simulink model "NPC_ANPC_Final_A"  (R2022b)
settings: Solver=ode4  StartTime=0.0  StopTime=1  FixedStep=1e-6  MaxStep=1e-4  RelTol=1e-3
InitFcn:
  | v=3000
  | r=0.000001
  | c=1000e-6
  | l=314
  | i=1000
  | r1=1000
  | t=1/3000
  | ma=2
  | f=2*pi*50
  | p1=(2*pi)/3
  | p2=-(2*pi)/3
libraries: spsIGBTDiodeLib x25, spsDiodeLib x19, simulink x12, spsSeriesRLCBranchLib x7, spsVoltageMeasurementLib x3, spsCurrentMeasurementLib x2, spsMeanLib x2, spspowerguiLib x2, spsPermanentMagnetSynchronousMachineLib x1, spsThreePhaseVIMeasurementLib x1, spsWindTurbineLib x1
settings Model: Creator=dell  LastModifiedBy=shubh
settings SolverCC: AlgebraicLoopSolver=TrustRegion
settings DataIOCC: ReturnWorkspaceOutputs=off
settings DebuggingCC: UnconnectedInputMsg=warning  UnconnectedOutputMsg=warning  UnconnectedLineMsg=warning  SFMachineParentedDataDiag=warning  ArithmeticOperatorsInVariantConditions=warning
settings ModelReferenceCC: EnableRefExpFcnMdlSchedulingChecks=on
settings SFSimCC: SimUseLocalCustomCode=off  CustomCodeUndefinedFunction=UseInterfaceOnly
settings RTWCC: RTWUseLocalCustomCode=off
settings CodeAppCC: StateflowObjectComments=on
settings SimscapeCC: SimscapeNormalizeSystem=off

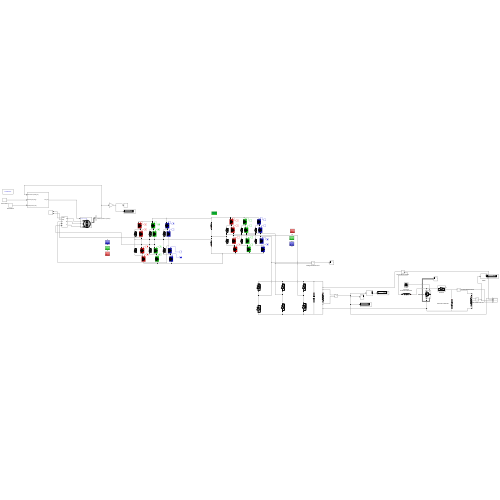
[thumbnail: Simulink's stored preview of the top-level diagram]
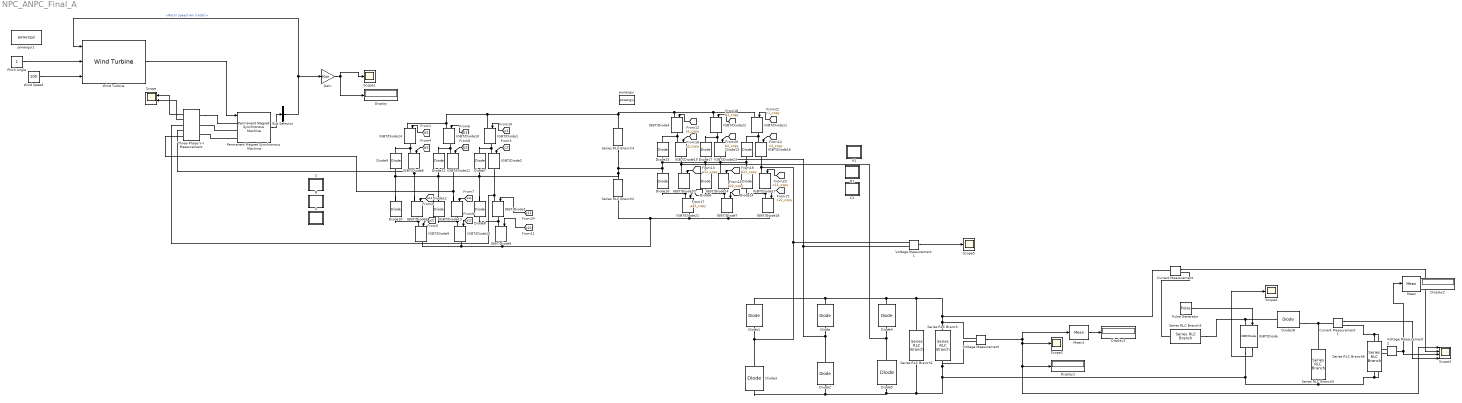
== system NPC_ANPC_Final_A ==
  A : Subsystem
  A1 : Subsystem
  B : Subsystem
  B1 : Subsystem
  Bus Selector : BusSelector  OutputSignals=Rotor speed wm (rad/s)
  C : Subsystem
  C1 : Subsystem
  Current Measurement : spsCurrentMeasurementLib/Current Measurement  PhasorSimulation=off  OutputType=Complex  PSBequivalent=0
  Current Measurement1 : spsCurrentMeasurementLib/Current Measurement  PhasorSimulation=off  OutputType=Complex  PSBequivalent=0
  Diode{,1..17} (18 alike) : spsDiodeLib/Diode  Ron=0.001  Lon=0  Vf=0.8  IC=0  UseSnubber=0  Rs=500  Cs=250e-9  Measurements=off
  Diode18 : spsDiodeLib/Diode  Ron=0.001  Lon=0  Vf=0.8  IC=0  UseSnubber=0  Rs=500  Cs=250e-9  Measurements=on
  Display{,1..3} (4 alike) : Display
  Gain : Gain  Gain=30/pi
  IGBT/Diode : spsIGBTDiodeLib/IGBT//Diode  Ron=1e-3  Rs=1e5  Cs=inf  Measurements=on
  IGBT/Diode{1..24} (24 alike) : spsIGBTDiodeLib/IGBT//Diode  Ron=1e-3  Rs=1e5  Cs=inf  Measurements=off
  Mean : spsMeanLib/Mean  Freq=60  Vinit=0  Ts=0
  Mean1 : spsMeanLib/Mean  Freq=60  Vinit=0  Ts=0
  Permanent Magnet Synchronous Machine : spsPermanentMagnetSynchronousMachineLib/Permanent Magnet Synchronous Machine  NbPhases=3  FluxDistribution=Sinusoidal  RotorType=Round  MechanicalLoad=Torque Tm  PresetModel=No  ShowDetailedParameters=on  MeasurementBus=off  Resistance=0.0485  Inductance=8.5e-3  dqInductances=[8.5e-3,8.5e-3]  La=0.000395  MachineConstant=Flux linkage established by magnets (V.s)  Flux=0.1194  VoltageCst=86.6271  TorqueCst=0.7164  Flat=120  Mechanical=[0.0027 0.0004924 4 0]  PolePairs=4  InitialConditions=[0,0, 0,0]  InitialConditions5ph=[0 0 0 0 0 0]  RefAngle=90 degrees behind phase A axis (modified Park)  IterativeDiscreteModel=Trapezoidal non iterative  TsBlock=-1  TsPowergui=0
  Pitch Angle : Constant
  Pulse Generator : DiscretePulseGenerator  PulseType=Time based  Amplitude=4  Period=1/5000  PulseWidth=60
  Scope : Scope  NumInputPorts=2
  Scope{1..2,4..5} (4 alike) : Scope
  Scope3 : Scope  NumInputPorts=4
  Series RLC Branch : spsSeriesRLCBranchLib/Series RLC Branch  LConnTagsString=__new0  RConnTagsString=__new0  BranchType=R  Resistance=10  Inductance=1e-3  SetiL0=off  InitialCurrent=0  Capacitance=1e-6  Setx0=off  InitialVoltage=0  Measurements=None
  Series RLC Branch1 : spsSeriesRLCBranchLib/Series RLC Branch  LConnTagsString=__new0  RConnTagsString=__new0  BranchType=C  Resistance=10  Inductance=10e-3  SetiL0=off  InitialCurrent=0  Capacitance=10e-3  Setx0=off  InitialVoltage=0  Measurements=None
  Series RLC Branch2 : spsSeriesRLCBranchLib/Series RLC Branch  LConnTagsString=__new0  RConnTagsString=__new0  BranchType=C  Resistance=1  Inductance=1e-3  SetiL0=off  InitialCurrent=0  Capacitance=5000e-6  Setx0=off  InitialVoltage=i  Measurements=None
  Series RLC Branch3 : spsSeriesRLCBranchLib/Series RLC Branch  LConnTagsString=__new0  RConnTagsString=__new0  BranchType=L  Resistance=1  Inductance=6e-3  SetiL0=off  InitialCurrent=0  Capacitance=1e-6  Setx0=off  InitialVoltage=0  Measurements=None
  Series RLC Branch4 : spsSeriesRLCBranchLib/Series RLC Branch  LConnTagsString=__new0  RConnTagsString=__new0  BranchType=C  Resistance=1  Inductance=1e-3  SetiL0=off  InitialCurrent=0  Capacitance=5000e-6  Setx0=off  InitialVoltage=i  Measurements=None
  Series RLC Branch5 : spsSeriesRLCBranchLib/Series RLC Branch  LConnTagsString=__new0  RConnTagsString=__new0  BranchType=C  Resistance=1  Inductance=6e-3  SetiL0=off  InitialCurrent=0  Capacitance=5000e-6  Setx0=off  InitialVoltage=0  Measurements=None
  Series RLC Branch6 : spsSeriesRLCBranchLib/Series RLC Branch  LConnTagsString=__new0  RConnTagsString=__new0  BranchType=R  Resistance=12.5  Inductance=6e-3  SetiL0=off  InitialCurrent=0  Capacitance=1e-6  Setx0=off  InitialVoltage=0  Measurements=None
  Three-Phase V-I Measurement : spsThreePhaseVIMeasurementLib/Three-Phase V-I Measurement  VoltageMeasurement=phase-to-phase  SetLabelV=off  LabelV=Vabc  Vpu=off  VpuLL=off  CurrentMeasurement=yes  SetLabelI=off  LabelI=Iabc  Ipu=off  Pbase=100e6  Vbase=500e3  OutputType=Complex  PhasorSimulation=off  PSBequivalent=0
  Voltage Measurement : spsVoltageMeasurementLib/Voltage Measurement  PhasorSimulation=off  OutputType=Complex  PSBequivalent=0
  Voltage Measurement1 : spsVoltageMeasurementLib/Voltage Measurement  PhasorSimulation=off  OutputType=Complex  PSBequivalent=0
  Voltage Measurement2 : spsVoltageMeasurementLib/Voltage Measurement  PhasorSimulation=off  OutputType=Complex  PSBequivalent=0
  Wind Speed : Constant  Value=100
  Wind Turbine : spsWindTurbineLib/Wind Turbine  Pnom=1.5e6  Pelec_base=1.5e6/0.9  wind_base=12  P_wind_base=0.73  speed_nom=1.2  pitch_angle=0  c1_c6="[0.51763          116          0.4            5           21     0.006795]"  cp_nom=0.48  lambda_nom=8.1
  powergui : spspowerguiLib/powergui  Priority=1  SimulationMode=Discrete  SampleTime=1e-6  frequency=60  Iterations=50  frequencyindice=0  Pbase=100e6  ErrMax=1e-4  UnitsV=kV  UnitsW=MW  buscounter=0  FunctionMessages=off  echomessages=off  EnableUseOfTLC=off  CurrentSourceSwitches=off  DisableSnubberDevices=off  DisableRonSwitches=off  DisableVfSwitches=off  DisplayEquations=off  AutomaticDiscreteSolvers=off  SolverType=Tustin/Backward Euler (TBE)  Interpol=off  ExternalGateDelay=off  methode=off  Ts=100  x0status=blocks  SPID=on  SwTol=0  HookPort=off  NonlinearTolerance=1e-4  nMaxIteration=100  ContinueOnMaxIteration=off  RestoreLinks=warning  ResistiveCurrentMeasurement=off  Frange=[0:2:500]  Ylog=off  Xlog=on  ShowGrid=off  save=off  variable=ZData  structure=d  ZoomFFT=off  StartTime=0.2  cycles=2  DisplayStyle=1  fundamental=50  FreqAxis=on  MaxFrequency=40000  frequencyindicesteady=1  RmsSteady=1  display=off
  powergui1 : spspowerguiLib/powergui  Priority=1  SimulationMode=Continuous  SampleTime=50e-6  frequency=60  Iterations=50  frequencyindice=0  Pbase=100e6  ErrMax=1e-4  UnitsV=kV  UnitsW=MW  buscounter=0  FunctionMessages=off  echomessages=off  EnableUseOfTLC=off  CurrentSourceSwitches=off  DisableSnubberDevices=off  DisableRonSwitches=off  DisableVfSwitches=off  DisplayEquations=off  AutomaticDiscreteSolvers=off  SolverType=Tustin/Backward Euler (TBE)  Interpol=off  ExternalGateDelay=off  methode=off  Ts=100  x0status=blocks  SPID=on  SwTol=0  HookPort=off  NonlinearTolerance=1e-4  nMaxIteration=100  ContinueOnMaxIteration=off  RestoreLinks=warning  ResistiveCurrentMeasurement=off  Frange=[0:2:500]  Ylog=off  Xlog=on  ShowGrid=off  save=off  variable=ZData  structure=0  ZoomFFT=off  StartTime=0.0  cycles=1  DisplayStyle=1  fundamental=60  FreqAxis=off  MaxFrequency=1000  frequencyindicesteady=1  RmsSteady=1  display=off
  wires:
  Gain/1 -> Display/1, Scope1/1
  Pitch Angle/1 -> Wind Turbine/2
  Bus Selector/1 -> Gain/1, Wind Turbine/1  "<Rotor speed wm (rad/s)>"
  Three-Phase V-I Measurement/1 -> Scope/1
  Wind Turbine/1 -> Permanent Magnet Synchronous Machine/1
  Permanent Magnet Synchronous Machine/1 -> Bus Selector/1
  Wind Speed/1 -> Wind Turbine/3
  Three-Phase V-I Measurement/2 -> Scope/2
  [c22_copy] -> IGBT/Diode18/1
  [c2_copy] -> IGBT/Diode16/1
  [c1_copy] -> IGBT/Diode11/1
  [c11_copy] -> IGBT/Diode17/1
  [b22_copy] -> IGBT/Diode7/1
  [b11_copy] -> IGBT/Diode24/1
  [b2_copy] -> IGBT/Diode23/1
  [b1_copy] -> IGBT/Diode22/1
  [a22_copy] -> IGBT/Diode21/1
  [a11_copy] -> IGBT/Diode20/1
  [a2_copy] -> IGBT/Diode19/1
  [a1_copy] -> IGBT/Diode4/1
  [c1] -> IGBT/Diode1/1
  [c2] -> IGBT/Diode2/1
  [c22] -> IGBT/Diode5/1
  [a22] -> IGBT/Diode9/1
  [a2] -> IGBT/Diode6/1
  [a11] -> IGBT/Diode8/1
  [b2] -> IGBT/Diode12/1
  [b1] -> IGBT/Diode10/1
  [b11] -> IGBT/Diode13/1
  [b22] -> IGBT/Diode15/1
  [c11] -> IGBT/Diode3/1
  [a1] -> IGBT/Diode14/1
  Voltage Measurement1/1 -> Scope5/1
  Mean/1 -> Display2/1
  IGBT/Diode/1 -> Scope4/1
  Pulse Generator/1 -> IGBT/Diode/1
  Voltage Measurement2/1 -> Mean/1, Scope3/3
  Mean1/1 -> Display3/1
  Current Measurement1/1 -> Scope3/4
  Current Measurement/1 -> Scope3/2
  Voltage Measurement/1 -> Scope3/1, Display1/1, Scope2/1, Mean1/1
  connections:
  Permanent Magnet Synchronous Machine/LConn2 -- Three-Phase V-I Measurement/LConn2
  Three-Phase V-I Measurement/LConn1 -- Permanent Magnet Synchronous Machine/LConn1
  Permanent Magnet Synchronous Machine/LConn3 -- Three-Phase V-I Measurement/LConn3
  IGBT/Diode19/LConn1 -- Diode15/RConn1 -- IGBT/Diode4/RConn1
  IGBT/Diode21/LConn1 -- Diode16/LConn1 -- IGBT/Diode20/RConn1
  IGBT/Diode23/LConn1 -- Diode17/RConn1 -- IGBT/Diode22/RConn1
  IGBT/Diode7/LConn1 -- Diode6/LConn1 -- IGBT/Diode24/RConn1
  IGBT/Diode16/LConn1 -- Diode13/RConn1 -- IGBT/Diode11/RConn1
  IGBT/Diode18/LConn1 -- Diode14/LConn1 -- IGBT/Diode17/RConn1
  Diode12/RConn1 -- Diode11/LConn1 -- Diode10/RConn1 -- Diode9/LConn1 -- Diode7/LConn1 -- Series RLC Branch4/LConn1 -- Diode16/RConn1 -- Diode15/LConn1 -- Diode6/RConn1 -- Diode17/LConn1 -- Diode14/RConn1 -- Diode13/LConn1 -- Series RLC Branch2/RConn1 -- Diode8/RConn1
  IGBT/Diode24/LConn1 -- IGBT/Diode23/RConn1 -- Voltage Measurement1/LConn2 -- Diode/LConn1 -- Diode2/RConn1
  IGBT/Diode15/RConn1 -- IGBT/Diode9/RConn1 -- IGBT/Diode5/RConn1 -- Series RLC Branch2/LConn1 -- IGBT/Diode21/RConn1 -- IGBT/Diode7/RConn1 -- IGBT/Diode18/RConn1
  IGBT/Diode10/LConn1 -- IGBT/Diode14/LConn1 -- IGBT/Diode1/LConn1 -- Series RLC Branch4/RConn1 -- IGBT/Diode4/LConn1 -- IGBT/Diode22/LConn1 -- IGBT/Diode11/LConn1
  Diode4/LConn1 -- IGBT/Diode20/LConn1 -- IGBT/Diode19/RConn1 -- Diode5/RConn1
  Diode8/LConn1 -- IGBT/Diode5/LConn1 -- IGBT/Diode3/RConn1
  Diode10/LConn1 -- IGBT/Diode9/LConn1 -- IGBT/Diode8/RConn1
  Diode12/LConn1 -- IGBT/Diode15/LConn1 -- IGBT/Diode13/RConn1
  IGBT/Diode14/RConn1 -- IGBT/Diode6/LConn1 -- Diode9/RConn1
  Diode11/RConn1 -- IGBT/Diode12/LConn1 -- IGBT/Diode10/RConn1
  Diode7/RConn1 -- IGBT/Diode2/LConn1 -- IGBT/Diode1/RConn1
  Three-Phase V-I Measurement/RConn1 -- IGBT/Diode3/LConn1 -- IGBT/Diode2/RConn1
  Series RLC Branch1/RConn1 -- Voltage Measurement/LConn2 -- Series RLC Branch/RConn1 -- Voltage Measurement2/LConn2 -- Series RLC Branch6/RConn1 -- Series RLC Branch5/RConn1 -- IGBT/Diode/RConn1 -- Diode5/LConn1 -- Diode3/LConn1 -- Diode2/LConn1
  Diode18/LConn1 -- Series RLC Branch3/LConn1 -- IGBT/Diode/LConn1
  Diode4/RConn1 -- Voltage Measurement/LConn1 -- Series RLC Branch/LConn1 -- Current Measurement/LConn1 -- Series RLC Branch1/LConn1 -- Diode1/RConn1 -- Diode/RConn1
  Series RLC Branch6/LConn1 -- Voltage Measurement2/LConn1 -- Current Measurement1/RConn1
  Current Measurement1/LConn1 -- Diode18/RConn1 -- Series RLC Branch5/LConn1
  Series RLC Branch3/RConn1 -- Current Measurement/RConn1
  IGBT/Diode13/LConn1 -- IGBT/Diode12/RConn1 -- Three-Phase V-I Measurement/RConn3
  IGBT/Diode8/LConn1 -- Three-Phase V-I Measurement/RConn2 -- IGBT/Diode6/RConn1
  Voltage Measurement1/LConn1 -- Diode1/LConn1 -- Diode3/RConn1 -- IGBT/Diode17/LConn1 -- IGBT/Diode16/RConn1

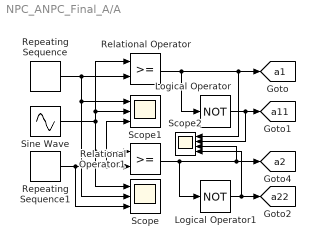
== system NPC_ANPC_Final_A/A ==
  Logical Operator : Logic  Operator=NOT  AllPortsSameDT=off  OutDataTypeStr=boolean
  Logical Operator1 : Logic  Operator=NOT  AllPortsSameDT=off  OutDataTypeStr=boolean
  Relational Operator : RelationalOperator  OutDataTypeStr=boolean  RndMeth=Simplest  InputSameDT=off
  Relational Operator1 : RelationalOperator  OutDataTypeStr=boolean  RndMeth=Simplest  InputSameDT=off
  Repeating Sequence : simulink/Sources/Repeating Sequence  rep_seq_t=[0 t/2 t]  rep_seq_y=[0 2 0]
  Repeating Sequence1 : simulink/Sources/Repeating Sequence  rep_seq_t=[0 t/2 t]  rep_seq_y=[-2 0 -2]
  Scope : Scope  NumInputPorts=3
  Scope1 : Scope  NumInputPorts=3
  Scope2 : Scope  NumInputPorts=4
  Sine Wave : Sin  Amplitude=ma  Frequency=f  SampleTime=0
  tag scope: a11=global, a1=global, a22=global, a2=global
  wires:
  Sine Wave/1 -> Relational Operator/1, Scope1/2, Relational Operator1/1, Scope/1
  Relational Operator1/1 -> [a2], Scope2/3, Logical Operator1/1
  Relational Operator/1 -> Logical Operator/1, [a1], Scope2/1
  Repeating Sequence1/1 -> Relational Operator1/2, Scope1/3, Scope/3
  Repeating Sequence/1 -> Relational Operator/2, Scope/2, Scope1/1
  Logical Operator1/1 -> Scope2/4, [a22]
  Logical Operator/1 -> [a11], Scope2/2

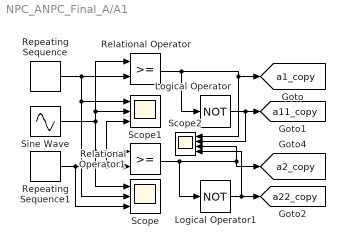
== system NPC_ANPC_Final_A/A1 ==
  Logical Operator : Logic  Operator=NOT  AllPortsSameDT=off  OutDataTypeStr=boolean
  Logical Operator1 : Logic  Operator=NOT  AllPortsSameDT=off  OutDataTypeStr=boolean
  Relational Operator : RelationalOperator  OutDataTypeStr=boolean  RndMeth=Simplest  InputSameDT=off
  Relational Operator1 : RelationalOperator  OutDataTypeStr=boolean  RndMeth=Simplest  InputSameDT=off
  Repeating Sequence : simulink/Sources/Repeating Sequence  rep_seq_t=[0 t/2 t]  rep_seq_y=[0 2 0]
  Repeating Sequence1 : simulink/Sources/Repeating Sequence  rep_seq_t=[0 t/2 t]  rep_seq_y=[-2 0 -2]
  Scope : Scope  NumInputPorts=3
  Scope1 : Scope  NumInputPorts=3
  Scope2 : Scope  NumInputPorts=4
  Sine Wave : Sin  Amplitude=ma  Frequency=f  SampleTime=0
  tag scope: a11_copy=global, a1_copy=global, a22_copy=global, a2_copy=global
  wires:
  Sine Wave/1 -> Relational Operator/1, Scope1/2, Relational Operator1/1, Scope/1
  Relational Operator1/1 -> [a2_copy], Scope2/3, Logical Operator1/1
  Relational Operator/1 -> Logical Operator/1, [a1_copy], Scope2/1
  Repeating Sequence1/1 -> Relational Operator1/2, Scope1/3, Scope/3
  Repeating Sequence/1 -> Relational Operator/2, Scope/2, Scope1/1
  Logical Operator1/1 -> Scope2/4, [a22_copy]
  Logical Operator/1 -> [a11_copy], Scope2/2

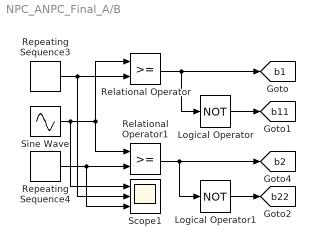
== system NPC_ANPC_Final_A/B ==
  Logical Operator : Logic  Operator=NOT  AllPortsSameDT=off  OutDataTypeStr=boolean
  Logical Operator1 : Logic  Operator=NOT  AllPortsSameDT=off  OutDataTypeStr=boolean
  Relational Operator : RelationalOperator  OutDataTypeStr=boolean  RndMeth=Simplest  InputSameDT=off
  Relational Operator1 : RelationalOperator  OutDataTypeStr=boolean  RndMeth=Simplest  InputSameDT=off
  Repeating Sequence3 : simulink/Sources/Repeating Sequence  rep_seq_t=[0 t/2 t]  rep_seq_y=[0 2 0]
  Repeating Sequence4 : simulink/Sources/Repeating Sequence  rep_seq_t=[0 t/2 t]  rep_seq_y=[-2 0 -2]
  Scope1 : Scope  NumInputPorts=3
  Sine Wave : Sin  Amplitude=ma  Frequency=f  Phase=p2  SampleTime=0
  tag scope: b11=global, b1=global, b22=global, b2=global
  wires:
  Logical Operator/1 -> [b11]
  Relational Operator/1 -> [b1], Logical Operator/1
  Relational Operator1/1 -> [b2], Logical Operator1/1
  Sine Wave/1 -> Relational Operator/1, Relational Operator1/1, Scope1/1
  Repeating Sequence4/1 -> Relational Operator1/2, Scope1/3
  Repeating Sequence3/1 -> Relational Operator/2, Scope1/2
  Logical Operator1/1 -> [b22]

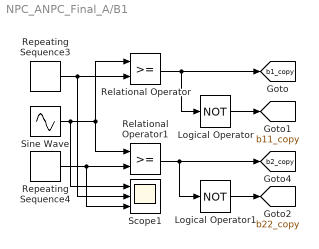
== system NPC_ANPC_Final_A/B1 ==
  Logical Operator : Logic  Operator=NOT  AllPortsSameDT=off  OutDataTypeStr=boolean
  Logical Operator1 : Logic  Operator=NOT  AllPortsSameDT=off  OutDataTypeStr=boolean
  Relational Operator : RelationalOperator  OutDataTypeStr=boolean  RndMeth=Simplest  InputSameDT=off
  Relational Operator1 : RelationalOperator  OutDataTypeStr=boolean  RndMeth=Simplest  InputSameDT=off
  Repeating Sequence3 : simulink/Sources/Repeating Sequence  rep_seq_t=[0 t/2 t]  rep_seq_y=[0 2 0]
  Repeating Sequence4 : simulink/Sources/Repeating Sequence  rep_seq_t=[0 t/2 t]  rep_seq_y=[-2 0 -2]
  Scope1 : Scope  NumInputPorts=3
  Sine Wave : Sin  Amplitude=ma  Frequency=f  Phase=p2  SampleTime=0
  tag scope: b11_copy=global, b1_copy=global, b22_copy=global, b2_copy=global
  wires:
  Logical Operator/1 -> [b11_copy]
  Relational Operator/1 -> [b1_copy], Logical Operator/1
  Relational Operator1/1 -> [b2_copy], Logical Operator1/1
  Sine Wave/1 -> Relational Operator/1, Relational Operator1/1, Scope1/1
  Repeating Sequence4/1 -> Relational Operator1/2, Scope1/3
  Repeating Sequence3/1 -> Relational Operator/2, Scope1/2
  Logical Operator1/1 -> [b22_copy]

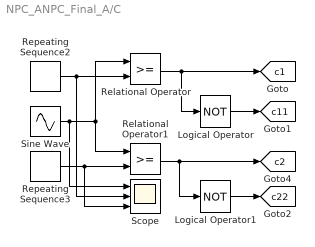
== system NPC_ANPC_Final_A/C ==
  Logical Operator : Logic  Operator=NOT  AllPortsSameDT=off  OutDataTypeStr=boolean
  Logical Operator1 : Logic  Operator=NOT  AllPortsSameDT=off  OutDataTypeStr=boolean
  Relational Operator : RelationalOperator  OutDataTypeStr=boolean  RndMeth=Simplest  InputSameDT=off
  Relational Operator1 : RelationalOperator  OutDataTypeStr=boolean  RndMeth=Simplest  InputSameDT=off
  Repeating Sequence2 : simulink/Sources/Repeating Sequence  rep_seq_t=[0 t/2 t]  rep_seq_y=[0 2 0]
  Repeating Sequence3 : simulink/Sources/Repeating Sequence  rep_seq_t=[0 t/2 t]  rep_seq_y=[-2 0 -2]
  Scope : Scope  NumInputPorts=3
  Sine Wave : Sin  Amplitude=ma  Frequency=f  Phase=p1  SampleTime=0
  tag scope: c11=global, c1=global, c22=global, c2=global
  wires:
  Logical Operator/1 -> [c11]
  Relational Operator/1 -> [c1], Logical Operator/1
  Relational Operator1/1 -> [c2], Logical Operator1/1
  Sine Wave/1 -> Relational Operator/1, Relational Operator1/1, Scope/1
  Repeating Sequence3/1 -> Relational Operator1/2, Scope/3
  Repeating Sequence2/1 -> Relational Operator/2, Scope/2
  Logical Operator1/1 -> [c22]

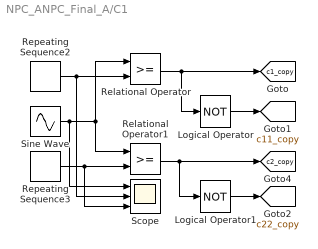
== system NPC_ANPC_Final_A/C1 ==
  Logical Operator : Logic  Operator=NOT  AllPortsSameDT=off  OutDataTypeStr=boolean
  Logical Operator1 : Logic  Operator=NOT  AllPortsSameDT=off  OutDataTypeStr=boolean
  Relational Operator : RelationalOperator  OutDataTypeStr=boolean  RndMeth=Simplest  InputSameDT=off
  Relational Operator1 : RelationalOperator  OutDataTypeStr=boolean  RndMeth=Simplest  InputSameDT=off
  Repeating Sequence2 : simulink/Sources/Repeating Sequence  rep_seq_t=[0 t/2 t]  rep_seq_y=[0 2 0]
  Repeating Sequence3 : simulink/Sources/Repeating Sequence  rep_seq_t=[0 t/2 t]  rep_seq_y=[-2 0 -2]
  Scope : Scope  NumInputPorts=3
  Sine Wave : Sin  Amplitude=ma  Frequency=f  Phase=p1  SampleTime=0
  tag scope: c11_copy=global, c1_copy=global, c22_copy=global, c2_copy=global
  wires:
  Logical Operator/1 -> [c11_copy]
  Relational Operator/1 -> [c1_copy], Logical Operator/1
  Relational Operator1/1 -> [c2_copy], Logical Operator1/1
  Sine Wave/1 -> Relational Operator/1, Relational Operator1/1, Scope/1
  Repeating Sequence3/1 -> Relational Operator1/2, Scope/3
  Repeating Sequence2/1 -> Relational Operator/2, Scope/2
  Logical Operator1/1 -> [c22_copy]
